simulink model "ineer_loop"  (R2022a)
settings: Solver=VariableStepAuto  StartTime=0.0  StopTime=10.0  RelTol=1e-3
undefined symbols (not defined in the file or in its folder): V_ref
libraries: cstblocks x4
settings Model: Creator=fcampreg  LastModifiedBy=fcampreg

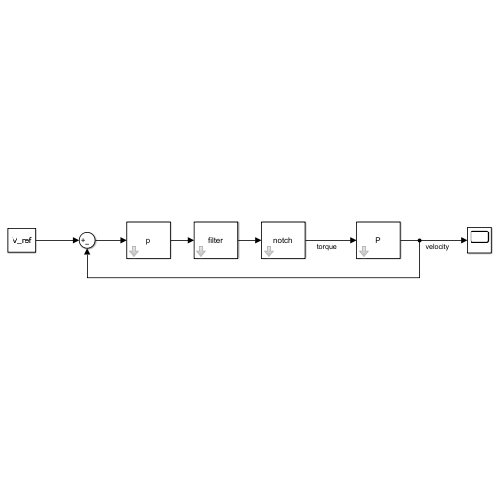
[thumbnail: Simulink's stored preview of the top-level diagram]
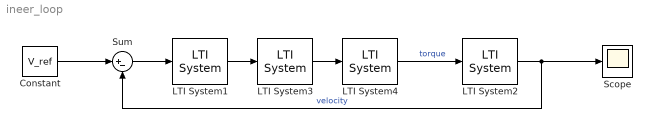
== system ineer_loop ==
  Constant : Constant  Value=V_ref
  LTI System1 : cstblocks/LTI System  sys=p  IC=[]
  LTI System2 : cstblocks/LTI System  sys=P  IC=[]
  LTI System3 : cstblocks/LTI System  sys=filter  IC=[]
  LTI System4 : cstblocks/LTI System  sys=notch  IC=[]
  Scope : Scope
  Sum : Sum  Inputs=|+-
  wires:
  LTI System1/1 -> LTI System3/1
  LTI System3/1 -> LTI System4/1
  LTI System4/1 -> LTI System2/1  "torque"
  LTI System2/1 -> Scope/1, Sum/2  "velocity"
  Sum/1 -> LTI System1/1
  Constant/1 -> Sum/1
